simulink model "DC_Motor_model_open_loop"  (R2026a)
settings: Solver=VariableStepAuto
model workspace (MAT data in the model file):
  B = Simulink.Parameter
  B.Value = 0.0001
  B.Complexity = 'real'
  B.Dimensions = [1 1]
  B.DataType = 'auto'
  J = Simulink.Parameter
  J.Value = 5e-05
  J.Complexity = 'real'
  J.Dimensions = [1 1]
  J.DataType = 'auto'
  Ke = Simulink.Parameter
  Ke.Value = 0.012
  Ke.Complexity = 'real'
  Ke.Dimensions = [1 1]
  Ke.DataType = 'auto'
  Kt = Simulink.Parameter
  Kt.Value = 0.012
  Kt.Complexity = 'real'
  Kt.Dimensions = [1 1]
  Kt.DataType = 'auto'
  L = Simulink.Parameter
  L.Value = 0.01
  L.Complexity = 'real'
  L.Dimensions = [1 1]
  L.DataType = 'auto'
  R = Simulink.Parameter
  R.Value = 5
  R.Complexity = 'real'
  R.Dimensions = [1 1]
  R.DataType = 'auto'
  TL = Simulink.Parameter
  TL.Value = 0
  TL.Complexity = 'real'
  TL.Dimensions = [1 1]
  TL.DataType = 'auto'

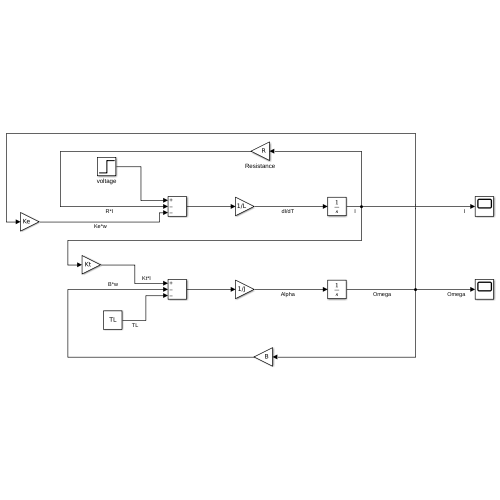
[thumbnail: Simulink's stored preview of the top-level diagram]
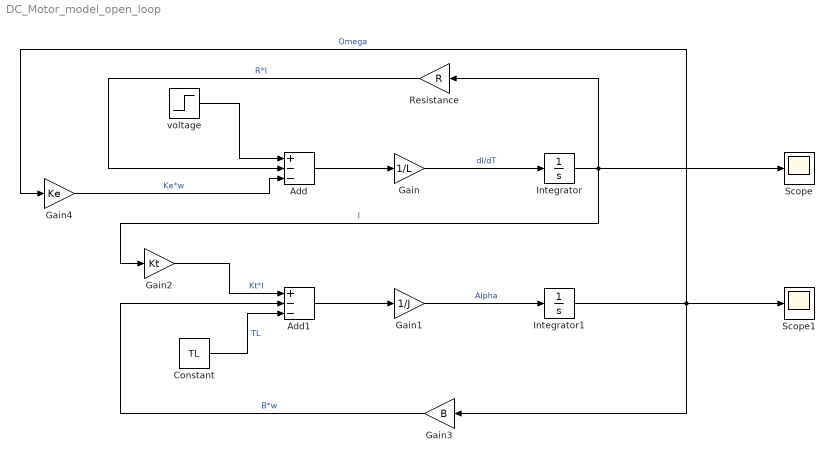
== system DC_Motor_model_open_loop ==
  Add : Sum  Inputs=+--
  Add1 : Sum  Inputs=+--
  Constant : Constant  Value=TL
  Gain : Gain  Gain=1/L
  Gain1 : Gain  Gain=1/J
  Gain2 : Gain  Gain=Kt
  Gain3 : Gain  Gain=B
  Gain4 : Gain  Gain=Ke
  Integrator : Integrator
  Integrator1 : Integrator
  Resistance : Gain  Gain=R
  Scope : Scope
      settings: ActiveDisplayYMinimum=-0.29789795118869822  ActiveDisplayYMaximum=2.6810815606982845
  Scope1 : Scope
      settings: ActiveDisplayYMinimum=-27.950460827084147  ActiveDisplayYMaximum=251.55414744375739
  voltage : Step  Time=0  FinalValue=12  SampleTime=0
  wires:
  Add/1 -> Gain/1
  Gain/1 -> Integrator/1  "dI/dT"
  Integrator/1 -> Resistance/1, Scope/1, Gain2/1  "I"
  Add1/1 -> Gain1/1
  Integrator1/1 -> Scope1/1, Gain4/1, Gain3/1  "Omega"
  Gain1/1 -> Integrator1/1  "Alpha"
  voltage/1 -> Add/1
  Resistance/1 -> Add/2  "R*I"
  Gain2/1 -> Add1/1  "Kt*I"
  Gain3/1 -> Add1/2  "B*w"
  Constant/1 -> Add1/3  "TL"
  Gain4/1 -> Add/3  "Ke*w"
